simulink model "model_R2020a"  (R2020a)
settings: Solver=FixedStepDiscrete  StartTime=0.0  StopTime=Inf  FixedStep=5e-3  RelTol=1e-3
values from neighbouring files (symbols this model uses):
  emin = 0.05    [simulate.m]
  gamma = 0.3    [simulate.m]
  k = 1    [simulate.m]
  omega_max = (pi/180)*300    (= 5.23598775598)    [simulate.m]
  u_max = 1.2    [simulate.m]
libraries: fuzblock x2, simulink x1
settings Model: Creator=mateu  LastModifiedBy=mateu
settings DebuggingCC: UnconnectedInputMsg=none  UnconnectedOutputMsg=none  UnconnectedLineMsg=none  SFMachineParentedDataDiag=error

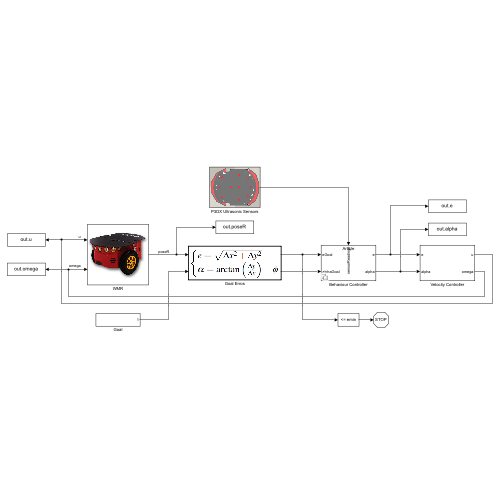
[thumbnail: Simulink's stored preview of the top-level diagram]
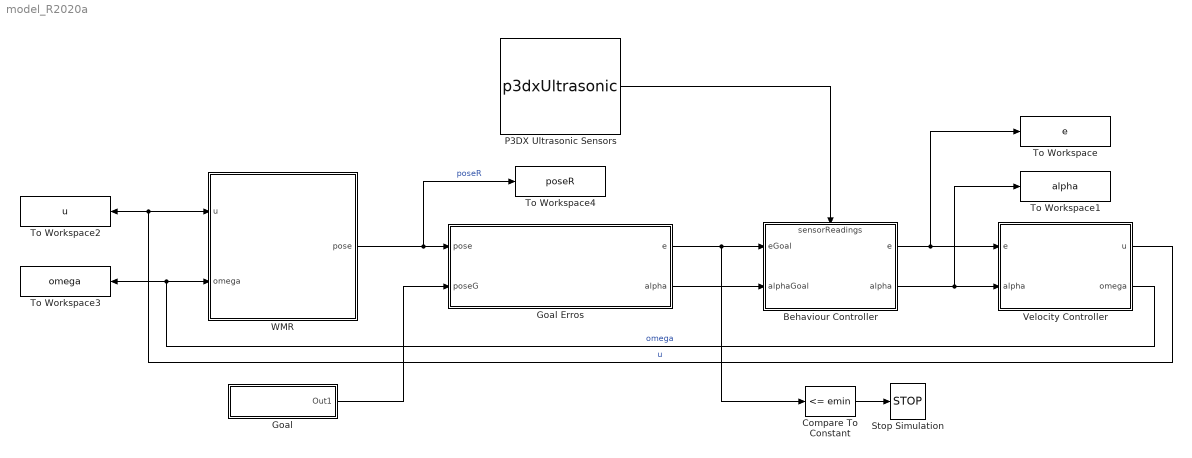
== system model_R2020a ==
  Behaviour Controller : Subsystem  Variant=on
      settings: PortSchema="{\"entries\":[{\"content\":{\"sides\":[{\"content\":{\"connectorIds\":[\"In1\",\"In2\"]},\"type\":\"ConnectorPlacement.EquallySpacedRectSide\",\"uuid\":\"213a18ad-7313-419c-8a71-2781d6b1397f\"},{\"content\":{\"connectorIds\":[\"Out1\",\"Out2\"],\"side\":\"RIGHT\"},\"type\":\"ConnectorPlacement.EquallySpacedRectSide\",\"uuid\":\"b99c4e5f-18e9-4fc0-9c68-3b156275d313\"},{\"content\":{\"connectorIds\":[\"In3\"],\"side\":\"TOP\"},\"type\":\"ConnectorPlacement.EquallySpacedRectSide\",\"uuid\":\"fd426b9d-f44a-424f-8de8-8f9078699f47\"}]},\"type\":\"ConnectorPlacement.EquallySpacedConnector\",\"uuid\":\"a0478f68-cb31-43be-ae4b-794c8a33903d\"}],\"packageUris\":[\"http://schema.mathworks.com/mf0/Connector/R2020b\"],\"version\":\"1.0\"}"
  Compare To Constant : simulink/Logic and Bit Operations/Compare To Constant  relop=<=  const=emin  OutDataTypeStr=boolean
  Goal : Subsystem  VariantControl=GOAL_COPPELIA
  Goal Erros : MATLAB Function  TreatAsAtomicUnit=on
  P3DX Ultrasonic Sensors : M-S-Function  FunctionName=p3dxUltrasonic
      mask Display: image('$imagefile'); % Use "Edit Image" on toolstrip to change.
  Stop Simulation : Stop
  To Workspace : ToWorkspace  VariableName=e  SaveFormat=Timeseries  SampleTime=-1
  To Workspace1 : ToWorkspace  VariableName=alpha  SaveFormat=Timeseries  SampleTime=-1
  To Workspace2 : ToWorkspace  VariableName=u  SaveFormat=Timeseries  SampleTime=-1
  To Workspace3 : ToWorkspace  VariableName=omega  SaveFormat=Timeseries  SampleTime=-1
  To Workspace4 : ToWorkspace  VariableName=poseR  SaveFormat=Timeseries  SampleTime=-1
  Velocity Controller : Subsystem
  WMR : Subsystem  VariantControl=UNICYCLE_COPPELIA
      mask Display: image('$imagefile'); % Use "Edit Image" on toolstrip to change.
  wires:
  WMR/1(pose) -> To Workspace4/1, Goal Erros/1(pose)  "poseR"
  Goal/1(Out1) -> Goal Erros/2(poseG)
  Compare To Constant/1 -> Stop Simulation/1
  Velocity Controller/1(u) -> WMR/1(u), To Workspace2/1  "u"
  Velocity Controller/2(omega) -> WMR/2(omega), To Workspace3/1  "omega"
  Goal Erros/1(e) -> Behaviour Controller/1(eGoal), Compare To Constant/1
  Goal Erros/2(alpha) -> Behaviour Controller/2(alphaGoal)
  P3DX Ultrasonic Sensors/1 -> Behaviour Controller/3(sensorReadings)
  Behaviour Controller/1(e) -> Velocity Controller/1(e), To Workspace/1
  Behaviour Controller/2(alpha) -> Velocity Controller/2(alpha), To Workspace1/1

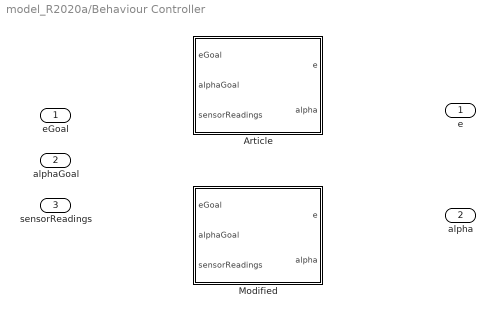
== system model_R2020a/Behaviour Controller ==
  eGoal : Inport
  alphaGoal : Inport  Port=2
  sensorReadings : Inport  Port=3
  Article : Subsystem  VariantControl=BC_ARTICLE
  Modified : Subsystem  VariantControl=BC_MODIFIED
  e : Outport
  alpha : Outport  Port=2

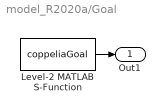
== system model_R2020a/Goal ==
  Level-2 MATLAB S-Function : M-S-Function  FunctionName=coppeliaGoal
  Out1 : Outport
  wires:
  Level-2 MATLAB S-Function/1 -> Out1/1

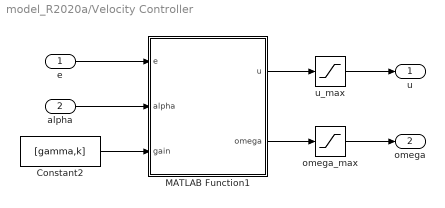
== system model_R2020a/Velocity Controller ==
  e : Inport
  alpha : Inport  Port=2
  Constant2 : Constant  Value=[gamma,k]
  MATLAB Function1 : MATLAB Function  TreatAsAtomicUnit=on
  omega_max : Saturate  UpperLimit=omega_max  LowerLimit=-omega_max
  u_max : Saturate  UpperLimit=u_max  LowerLimit=-u_max
  u : Outport
  omega : Outport  Port=2
  wires:
  Constant2/1 -> MATLAB Function1/3(gain)
  omega_max/1 -> omega/1
  u_max/1 -> u/1
  alpha/1 -> MATLAB Function1/2(alpha)
  e/1 -> MATLAB Function1/1(e)
  MATLAB Function1/2(omega) -> omega_max/1
  MATLAB Function1/1(u) -> u_max/1

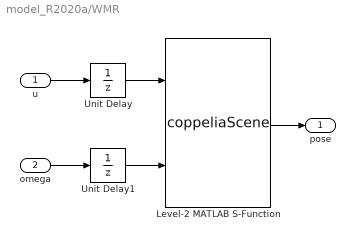
== system model_R2020a/WMR ==
  u : Inport
  omega : Inport  Port=2
  Level-2 MATLAB S-Function : M-S-Function  FunctionName=coppeliaScene
  Unit Delay : UnitDelay  SampleTime=-1  HasFrameUpgradeWarning=on
  Unit Delay1 : UnitDelay  SampleTime=-1  HasFrameUpgradeWarning=on
  pose : Outport
  wires:
  u/1 -> Unit Delay/1
  omega/1 -> Unit Delay1/1
  Level-2 MATLAB S-Function/1 -> pose/1
  Unit Delay/1 -> Level-2 MATLAB S-Function/1
  Unit Delay1/1 -> Level-2 MATLAB S-Function/2

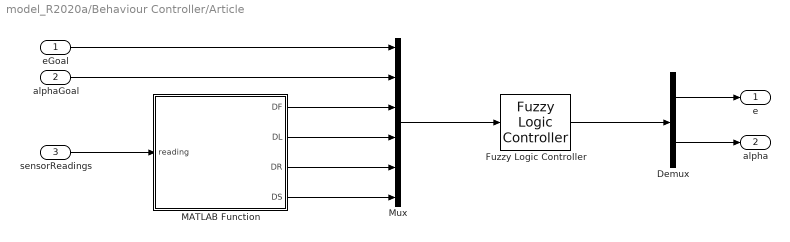
== system model_R2020a/Behaviour Controller/Article ==
  eGoal : Inport
  alphaGoal : Inport  Port=2
  sensorReadings : Inport  Port=3
  Demux : Demux  Outputs=2
  Fuzzy Logic Controller : fuzblock/Fuzzy Logic  Controller  FIS=fuzzyArticle  OutputSampleNumber=101  DataType=double  FuzzifiedInputs=off  RuleFiringStrengths=off  RuleOutputs=off  AggregatedOutputs=off  SimulateUsing=Interpreted execution  OutOfRangeInputValueMessage=warning  NoRuleFiredMessage=warning  EmptyOutputFuzzySetMessage=warning
  MATLAB Function : MATLAB Function  TreatAsAtomicUnit=on
  Mux : Mux  Inputs=6
  e : Outport
  alpha : Outport  Port=2
  wires:
  Fuzzy Logic Controller/1 -> Demux/1
  eGoal/1 -> Mux/1
  Mux/1 -> Fuzzy Logic Controller/1
  alphaGoal/1 -> Mux/2
  MATLAB Function/4(DS) -> Mux/6
  MATLAB Function/2(DL) -> Mux/4
  Demux/1 -> e/1
  Demux/2 -> alpha/1
  MATLAB Function/3(DR) -> Mux/5
  MATLAB Function/1(DF) -> Mux/3
  sensorReadings/1 -> MATLAB Function/1(reading)

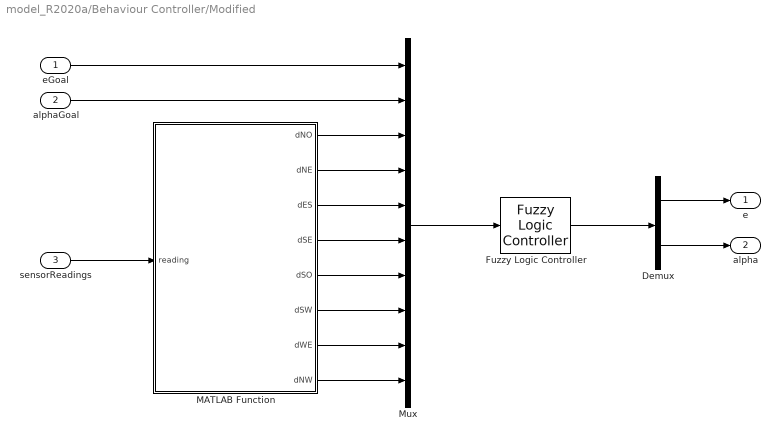
== system model_R2020a/Behaviour Controller/Modified ==
  eGoal : Inport
  alphaGoal : Inport  Port=2
  sensorReadings : Inport  Port=3
  Demux : Demux  Outputs=2
  Fuzzy Logic Controller : fuzblock/Fuzzy Logic  Controller  FIS=fuzzyModified  OutputSampleNumber=101  DataType=double  FuzzifiedInputs=off  RuleFiringStrengths=off  RuleOutputs=off  AggregatedOutputs=off  SimulateUsing=Interpreted execution  OutOfRangeInputValueMessage=warning  NoRuleFiredMessage=warning  EmptyOutputFuzzySetMessage=warning
  MATLAB Function : MATLAB Function  TreatAsAtomicUnit=on
  Mux : Mux  Inputs=10
  e : Outport
  alpha : Outport  Port=2
  wires:
  sensorReadings/1 -> MATLAB Function/1(reading)
  MATLAB Function/1(dNO) -> Mux/3
  MATLAB Function/2(dNE) -> Mux/4
  MATLAB Function/3(dES) -> Mux/5
  MATLAB Function/4(dSE) -> Mux/6
  MATLAB Function/5(dSO) -> Mux/7
  MATLAB Function/6(dSW) -> Mux/8
  MATLAB Function/7(dWE) -> Mux/9
  MATLAB Function/8(dNW) -> Mux/10
  alphaGoal/1 -> Mux/2
  eGoal/1 -> Mux/1
  Demux/2 -> alpha/1
  Demux/1 -> e/1
  Mux/1 -> Fuzzy Logic Controller/1
  Fuzzy Logic Controller/1 -> Demux/1

== matlab function model_R2020a/Behaviour Controller/Modified/MATLAB Function ==
  data: reading input; dNO output; dNE output; dES output; dSE output; dSO output; dSW output; dWE output; dNW output
function [dNO,dNE,dES,dSE,dSO,dSW,dWE,dNW] = getDistances(reading)

dNO = min(reading(4:5));
dNE = min(reading(6:7));
dES = min(reading(8:9));
dSE = min(reading(10:11));
dSO = min(reading(12:13));
dSW = min(reading(14:15));
dWE = min([reading(1),reading(16)]);
dNW = min(reading(2:3));

== matlab function model_R2020a/Goal Erros ==
  settings: updateMethod=DISCRETE  sampleTime=0.05
  data: pose input; e output; poseG input; alpha output
function [e,alpha] = errors(pose,poseG)

deltaX = poseG(1)-pose(1); deltaY = poseG(2)-pose(2);
phi = pose(3);

e = sqrt(deltaX^2 + deltaY^2);
alpha = atan2(deltaY,deltaX) - phi;

if alpha < -pi
    alpha = alpha + 2*pi;
elseif alpha >= pi
    alpha = alpha - 2*pi;
end

== matlab function model_R2020a/Velocity Controller/MATLAB Function1 ==
  settings: updateMethod=DISCRETE  sampleTime=0.05
  data: e input; u output; alpha input; omega output; gain input
function [u,omega] = control(e,alpha,gain)

gamma = gain(1); k = gain(2);

u = gamma*e*cos(alpha);
omega = k*alpha + gamma*cos(alpha)*sin(alpha);

== matlab function model_R2020a/Behaviour Controller/Article/MATLAB Function ==
  data: reading input; DF output; DL output; DR output; DS output
function [DF,DL,DR,DS] = getDistances(reading)

DF = min(reading(4:5)); 
DL = min(reading(1:15:end)); 
DR = min(reading(8:9));

if DR < DL
    DS = -DR;
else
    DS = DL;
end
